simulink model "stellaris_lp_print2"  (R2017a)
settings: Solver=ode3  StartTime=0.0  StopTime=10.0  FixedStep=0.1  RelTol=1e-3
libraries: stellaris_lp_lib x10, simulink x1
settings Model: ExtModeTrigDuration=2  Creator=peselnikmg  LastModifiedBy=Nilim
settings DataIOCC: LimitDataPoints=on  SaveFormat=Array  SignalLoggingSaveFormat=ModelDataLogs
settings OptimizationCC: PassReuseOutputArgsAs=Individual arguments  ExpressionDepthLimit=2147483647  MaxStackSize=64
settings DebuggingCC: ParameterTunabilityLossMsg=error  StateNameClashWarn=warning  SFUnexpectedBacktrackingDiag=warning  SFNoUnconditionalDefaultTransitionDiag=warning  SFExecutionAtInitializationDiag=none
settings HardwareCC: ProdBitPerPointer=32  ProdBitPerSizeT=32  ProdBitPerPtrDiffT=32  ProdLargestAtomicInteger=Long  ProdLargestAtomicFloat=Double  ProdWordSize=32  ProdHWDeviceType=ARM Compatible->ARM Cortex
settings ModelReferenceCC: PropagateSignalLabelsOutOfModel=off
settings SFSimCC: MATLABDynamicMemAlloc=off
settings RTWCC: SystemTargetFile=ert.tlc  HardwareBoard=Tiva TM4C123G Launchpad  TLCOptions=-aInlineSetEventsForThisBaseRateFcn=TLC_FALSE -aSuppressMultiTaskScheduler=TLC_FALSE -aRateBasedStepFcn=1  TemplateMakefile=ert_default_tmf  Description=Embedded Coder  GenerateReport=on  RTWVerbose=off  Toolchain=Texas Instruments Code Composer Studio (Tiva)  IncludeHyperlinkInReport=on  LaunchReport=on  GenerateTraceInfo=on  GenerateTraceReport=on  GenerateTraceReportSl=on  GenerateTraceReportSf=on  GenerateTraceReportEml=on
settings CodeAppCC: ForceParamTrailComments=on  IgnoreCustomStorageClasses=off  OperatorAnnotations=on  SimulinkDataObjDesc=on  SFDataObjDesc=on  MATLABFcnDesc=on  CustomSymbolStrType=$N$R$M  InsertBlockDesc=on  MATLABSourceComments=on  InternalIdentifier=Classic
settings ConfigComp: CovMetricSettings=dw  CovHtmlReporting=on  CovSaveCumulativeToWorkspaceVar=on  CovSaveSingleToWorkspaceVar=on  CovExternalEMLEnable=off

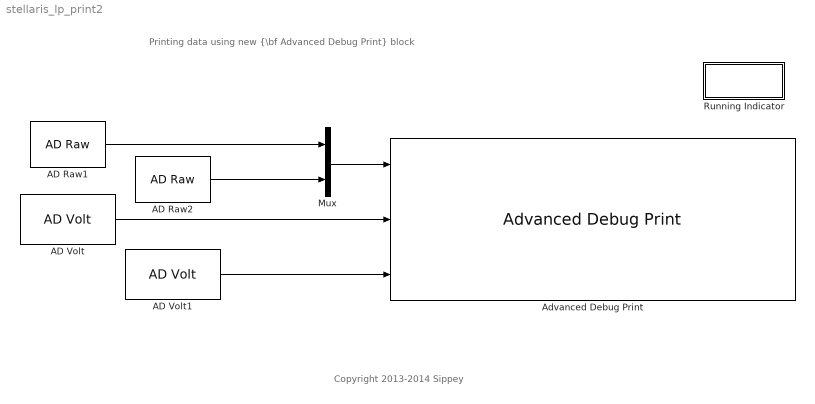
== system stellaris_lp_print2 ==
  note: Copyright 2013-2014 Sippey
  note: Printing data using new {\bf Advanced Debug Print} block
  AD Raw1 : stellaris_lp_lib/ADC/AD Raw  ch="1   PE3"  sample_time=0.1
      settings: SourceProductName=Run on Stellaris LaunchPad
  AD Raw2 : stellaris_lp_lib/ADC/AD Raw  ch="2   PE2"  sample_time=0.1
      settings: SourceProductName=Run on Stellaris LaunchPad
  AD Volt : stellaris_lp_lib/ADC/AD Volt  ch="3   PE1"  sample_time=0.1
      settings: SourceProductName=Run on Stellaris LaunchPad
  AD Volt1 : stellaris_lp_lib/ADC/AD Volt  ch="4   PE0"  sample_time=0.1
      settings: SourceProductName=Run on Stellaris LaunchPad
  Advanced Debug Print : stellaris_lp_lib/Debug/Advanced Debug Print  types={'uint32','single','double'}  fmt="'AD1 Raw=%4u, AD2 Raw=%04u,  AD3=%-7.3hf_V, AD4=%9.5f V\\r\\n'"  sample_time=0.1
      settings: SourceProductName=Run on Stellaris LaunchPad
  Mux : Mux  Inputs=2
  Running Indicator : Subsystem
  wires:
  AD Volt1/1 -> Advanced Debug Print/3
  Mux/1 -> Advanced Debug Print/1
  AD Raw1/1 -> Mux/1
  AD Raw2/1 -> Mux/2
  AD Volt/1 -> Advanced Debug Print/2

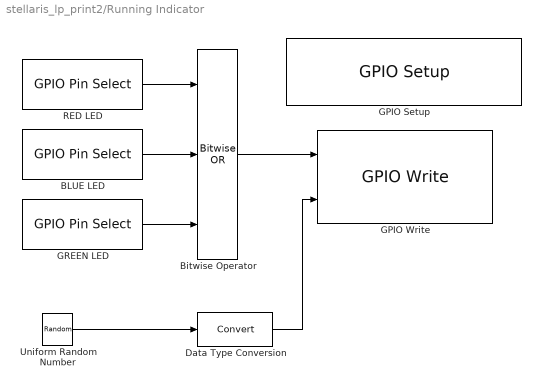
== system stellaris_lp_print2/Running Indicator ==
  BLUE LED : stellaris_lp_lib/GPIO/GPIO Pin Select  GPIO_PIN_X=GPIO_PIN_2
      settings: SourceProductName=Run on Stellaris LaunchPad
  Bitwise Operator : simulink/Logic and Bit Operations/Bitwise Operator  logicop=OR  UseBitMask=off  NumInputPorts=3  BitMask=bin2dec('11011001')  BitMaskRealWorld=Stored Integer
  Data Type Conversion : DataTypeConversion
  GPIO Setup : stellaris_lp_lib/GPIO/GPIO Setup  GPIO_PORTX_BASE=GPIO_PORTF_BASE  PinsOutput_0=Input  PinsOutput_1=Output  PinsOutput_2=Output  PinsOutput_3=Output  PinsOutput_4=Input  PinsOutput_5=Input  PinsOutput_6=Input  PinsOutput_7=Input
      settings: SourceProductName=Run on Stellaris LaunchPad
  GPIO Write : stellaris_lp_lib/GPIO/GPIO Write  GPIO_PORTX_BASE=GPIO_PORTF_BASE  SampleTime=-1
      settings: SourceProductName=Run on Stellaris LaunchPad
  GREEN LED : stellaris_lp_lib/GPIO/GPIO Pin Select  GPIO_PIN_X=GPIO_PIN_3
      settings: SourceProductName=Run on Stellaris LaunchPad
  RED LED : stellaris_lp_lib/GPIO/GPIO Pin Select  GPIO_PIN_X=GPIO_PIN_1
      settings: SourceProductName=Run on Stellaris LaunchPad
  Uniform Random Number : UniformRandomNumber  Minimum=2  Maximum=16  SampleTime=0.2
  wires:
  BLUE LED/1 -> Bitwise Operator/2
  RED LED/1 -> Bitwise Operator/1
  GREEN LED/1 -> Bitwise Operator/3
  Bitwise Operator/1 -> GPIO Write/1
  Uniform Random Number/1 -> Data Type Conversion/1
  Data Type Conversion/1 -> GPIO Write/2
